simulink model "arqSimModel"  (R2019a)
settings: Solver=VariableStepAuto  StartTime=0.0  StopTime=10.0  RelTol=1e-3
undefined symbols (not defined in the file or in its folder): WLAN
libraries: truetime x6
settings Model: Creator=Alvaro UAO  LastModifiedBy=Alvaro UAO

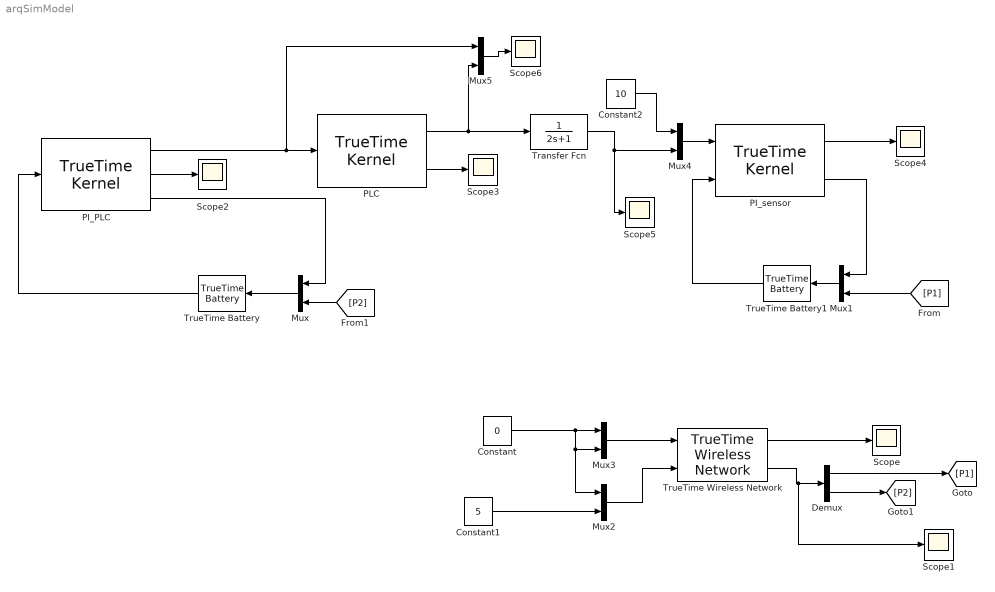
== system arqSimModel ==
  Constant : Constant  Value=0
  Constant1 : Constant  Value=5
  Constant2 : Constant  Value=10
  Demux : Demux  Outputs=2
  Mux{,1..5} (6 alike) : Mux  Inputs=2
  PI_PLC : truetime/TrueTime Kernel  sfun=PI_PLC_init  args=[]  ninputsoutputs=[0 1]  ntriggers=0  trigtype=falling  nwnodenbr=[2]  clockoffsetdrift=[0 0]  schedoutput=on  battery=on  poweroutput=on  label=1: 2
  PI_sensor : truetime/TrueTime Kernel  sfun=PI_Sensor_init  args=[]  ninputsoutputs=[2 0]  ntriggers=0  trigtype=falling  nwnodenbr=[1]  clockoffsetdrift=[0 0]  schedoutput=on  battery=on  poweroutput=on  label=1: 1
  PLC : truetime/TrueTime Kernel  sfun=plc_init  args=[]  ninputsoutputs=[1 1]  ntriggers=0  trigtype=falling  nwnodenbr=[]  clockoffsetdrift=[0 0]  schedoutput=on  battery=off  poweroutput=off
  Scope{,1..6} (7 alike) : Scope
  Transfer Fcn : TransferFcn  Denominator=[2 1]
  TrueTime Battery : truetime/TrueTime Battery  energy=1
  TrueTime Battery1 : truetime/TrueTime Battery  energy=1
  TrueTime Wireless Network : truetime/TrueTime Wireless  Network  nwtype=802.11b (WLAN)  nwnbr=1  nnodes=2  rate=800000  minsize=272  transpower=30  threshold=-48  use_pathloss_function=default  pathloss=3.5  acktimeout=0.00004  retrylimit=5  error_threshold=0.03  lossprob=0  seed=0  scheduleoutput=on  poweroutput=on
  wires:
  TrueTime Battery/1 -> PI_PLC/1
  PI_PLC/1 -> Mux5/1, PLC/1
  PI_PLC/3 -> Mux/1
  Mux/1 -> TrueTime Battery/1
  TrueTime Wireless Network/1 -> Scope/1
  TrueTime Wireless Network/2 -> Scope1/1, Demux/1
  Mux2/1 -> TrueTime Wireless Network/2
  Constant1/1 -> Mux2/2
  Constant/1 -> Mux2/1, Mux3/2, Mux3/1
  Mux3/1 -> TrueTime Wireless Network/1
  Demux/1 -> [P1]
  Demux/2 -> [P2]
  [P2] -> Mux/2
  PI_PLC/2 -> Scope2/1
  PLC/2 -> Scope3/1
  TrueTime Battery1/1 -> PI_sensor/2
  Mux1/1 -> TrueTime Battery1/1
  [P1] -> Mux1/2
  PI_sensor/2 -> Mux1/1
  PI_sensor/1 -> Scope4/1
  PLC/1 -> Mux5/2, Transfer Fcn/1
  Mux4/1 -> PI_sensor/1
  Mux5/1 -> Scope6/1
  Transfer Fcn/1 -> Mux4/2, Scope5/1
  Constant2/1 -> Mux4/1
